simulink model "isInBeam"  (R2013b)
settings: Solver=FixedStepDiscrete  StartTime=0.0  StopTime=10.0  RelTol=1e-3
settings Model: Creator=davendano  LastModifiedBy=davendano
settings OptimizationCC: InlineParams=on

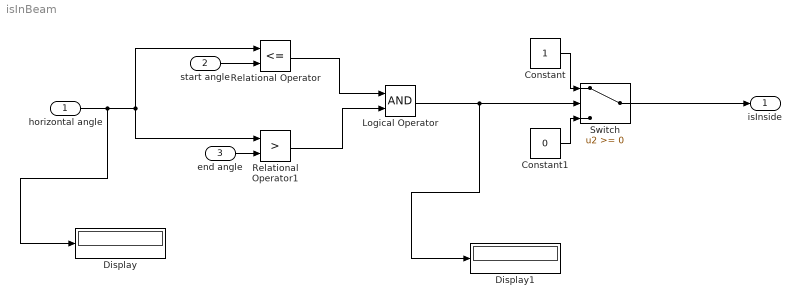
== system isInBeam ==
  horizontal angle : Inport
  start angle : Inport  Port=2
  end angle : Inport  Port=3
  Constant : Constant
  Constant1 : Constant  Value=0
  Display : Display
  Display1 : Display
  Logical Operator : Logic  AllPortsSameDT=off  OutDataTypeStr=boolean
  Relational Operator : RelationalOperator  Operator=<=  OutDataTypeStr=boolean
  Relational Operator1 : RelationalOperator  Operator=>  OutDataTypeStr=boolean
  Switch : Switch
  isInside : Outport
  wires:
  Constant/1 -> Switch/1
  Constant1/1 -> Switch/3
  Switch/1 -> isInside/1
  horizontal angle/1 -> Display/1, Relational Operator/1, Relational Operator1/1
  end angle/1 -> Relational Operator1/2
  start angle/1 -> Relational Operator/2
  Relational Operator/1 -> Logical Operator/1
  Relational Operator1/1 -> Logical Operator/2
  Logical Operator/1 -> Display1/1, Switch/2
